simulink model "arm_sim_pi_d_cont_nonlinear"  (R2022a)
settings: Solver=ode4  StartTime=0.0  StopTime=3  FixedStep=0.001  RelTol=1e-3
values from neighbouring files (symbols this model uses):
  dc = k*0.5    (= 2)    [arm_anime_pi_d_cont_nonlinear.m]    (also in plot_pi_d_cont_nonlinear_customize.m = k*0.5)
  kD = (alpha1*wm)/b0 - a1/b0 + a0/(alpha1*wm*b0)    [arm_anime_pi_d_cont_nonlinear.m]    (also in plot_pi_d_cont_nonlinear_customize.m)
  kI = (wm*a0)/(alpha1*b0)    [arm_anime_pi_d_cont_nonlinear.m]    (also in plot_pi_d_cont_nonlinear_customize.m)
  kP = wm^2/b0    [arm_anime_pi_d_cont_nonlinear.m]    (also in plot_pi_d_cont_nonlinear_customize.m)
  rc = k*30*(pi/180)    (= 2.09439510239)    [arm_anime_pi_d_cont_nonlinear.m]    (also in plot_pi_d_cont_nonlinear_customize.m = k*30*(pi/180))
undefined symbols (not defined in the file or in its folder): c, g, J, l, M
settings Model: Creator=kawata  LastModifiedBy=kawata
settings SolverCC: AlgebraicLoopSolver=TrustRegion
settings DataIOCC: ReturnWorkspaceOutputs=off
settings DebuggingCC: UnconnectedInputMsg=warning  UnconnectedOutputMsg=warning  UnconnectedLineMsg=warning  SFMachineParentedDataDiag=warning
settings RTWCC: DLArmComputeVersion=19.05

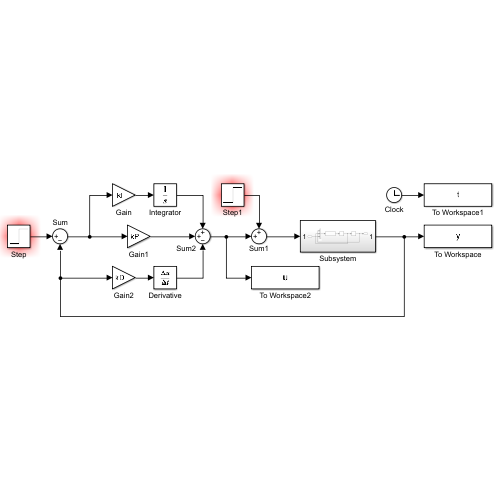
[thumbnail: Simulink's stored preview of the top-level diagram]
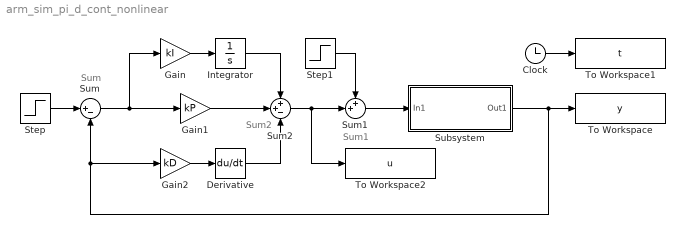
== system arm_sim_pi_d_cont_nonlinear ==
  note: Sum
  note: Sum1
  note: Sum2
  Clock : Clock
  Derivative : Derivative
  Gain : Gain  Gain=kI
  Gain1 : Gain  Gain=kP
  Gain2 : Gain  Gain=kD
  Integrator : Integrator
  Step : Step  Time=0  After=rc  SampleTime=0
  Step1 : Step  Time=1.5  After=dc  SampleTime=0
  Subsystem : Subsystem
  Sum : Sum  Inputs=|+-
  Sum1 : Sum  Inputs=++|
  Sum2 : Sum  Inputs=++-
  To Workspace : ToWorkspace  VariableName=y  SampleTime=-1
  To Workspace1 : ToWorkspace  VariableName=t  SampleTime=-1
  To Workspace2 : ToWorkspace  VariableName=u  SampleTime=-1
  wires:
  Step1/1 -> Sum1/1
  Sum2/1 -> To Workspace2/1, Sum1/2
  Sum1/1 -> Subsystem/1(In1)
  Integrator/1 -> Sum2/1
  Gain1/1 -> Sum2/2
  Derivative/1 -> Sum2/3
  Gain2/1 -> Derivative/1
  Sum/1 -> Gain/1, Gain1/1
  Gain/1 -> Integrator/1
  Step/1 -> Sum/1
  Subsystem/1(Out1) -> To Workspace/1, Gain2/1, Sum/2
  Clock/1 -> To Workspace1/1

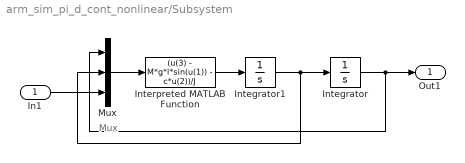
== system arm_sim_pi_d_cont_nonlinear/Subsystem ==
  note: Mux
  In1 : Inport
  Integrator : Integrator
  Integrator1 : Integrator
  Interpreted MATLAB Function : MATLABFcn  MATLABFcn=(u(3) - M*g*l*sin(u(1)) - c*u(2))/J
  Mux : Mux  Inputs=3
  Out1 : Outport  VectorParamsAs1DForOutWhenUnconnected=off
  wires:
  Integrator1/1 -> Mux/2, Integrator/1
  Integrator/1 -> Out1/1, Mux/1
  In1/1 -> Mux/3
  Interpreted MATLAB Function/1 -> Integrator1/1
  Mux/1 -> Interpreted MATLAB Function/1
